simulink model "Lab1_3rev2022A"  (R2022a)
settings: Solver=ode23tb  StartTime=0.0  StopTime=3  RelTol=1e-3
values from neighbouring files (symbols this model uses):
  ki = 700    [script1_3 (1).m]    (also in script1_3.m)
  kii = 600    [script1_3 (1).m]    (also in script1_3.m)
  kiv = 0.077471    [script1_3 (1).m]    (also in script1_3.m)
  kp = 2.93    [script1_3 (1).m]    (also in script1_3.m)
  kpi = 4    [script1_3 (1).m]    (also in script1_3.m)
  kpv = 0.0011508    [script1_3 (1).m]    (also in script1_3.m)
  L = 2e-3    (= 0.002)    [script1_3 (1).m]    (also in script1_3.m)
  w_ref = 2*pi*60    (= 376.991118431)    [script1_3 (1).m]    (also in script1_3.m)
libraries: spsIGBTDiodeLib x6, spsSeriesRLCBranchLib x4, simulink x3, spsPWMGenerator2LevelLib x3, spsdq0toabcLib x3, spsabctodq0Lib x2, spsPVArrayLib x1, spsPower3phInstantaneousLib x1, spsThreePhaseVIMeasurementLib x1, spsThreePhaseSourceLib x1, spsVoltageMeasurementLib x1, spspowerguiLib x1
settings Model: Creator=Daniel  LastModifiedBy=Daniel

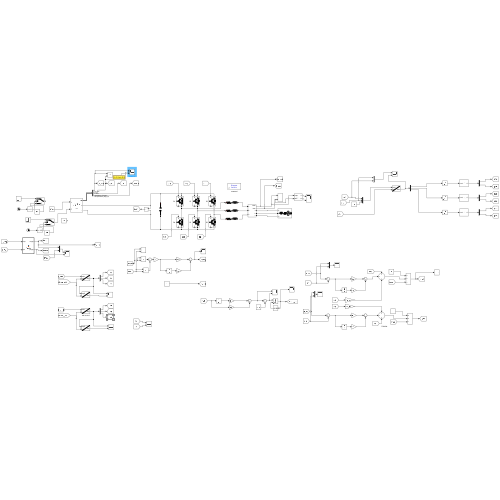
[thumbnail: Simulink's stored preview of the top-level diagram]
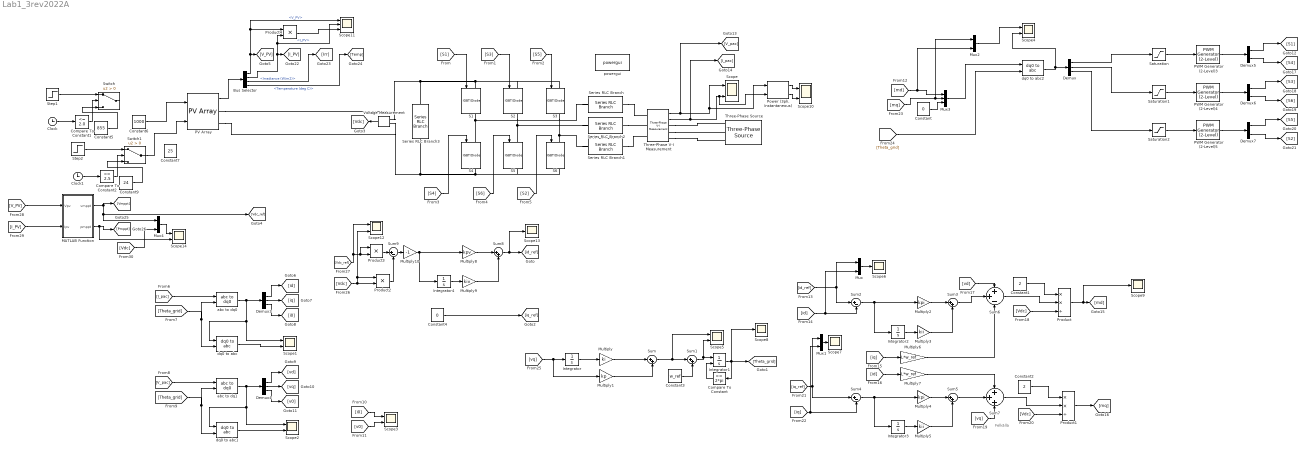
== system Lab1_3rev2022A ==
  note: Felkälla
  Bus Selector : BusSelector  OutputSignals=V_PV,I_PV,Irradiance (W/m2),Temperature (deg C)
  Clock : Clock
  Clock1 : Clock
  Compare To Constant : simulink/Logic and Bit Operations/Compare To Constant  relop=>=  const=2*pi  OutDataTypeStr=boolean
  Compare To Constant1 : simulink/Logic and Bit Operations/Compare To Constant  relop=<=  const=2.0  OutDataTypeStr=boolean
  Compare To Constant2 : simulink/Logic and Bit Operations/Compare To Constant  relop=<=  const=2.5  OutDataTypeStr=boolean
  Constant : Constant  Value=0
  Constant1 : Constant  Value=2
  Constant2 : Constant  Value=2
  Constant3 : Constant  Value=w_ref
  Constant4 : Constant  Value=0
  Constant5 : Constant  Value=855
  Constant6 : Constant  Value=1000
  Constant7 : Constant  Value=25
  Constant9 : Constant  Value=24
  Demux : Demux  Outputs=3
  Demux3 : Demux  Outputs=3
  Demux4 : Demux  Outputs=3
  Demux5 : Demux  Outputs=2
  Demux6 : Demux  Outputs=2
  Demux7 : Demux  Outputs=2
  Integrator{,2..4} (4 alike) : Integrator
  Integrator1 : Integrator  ExternalReset=rising
  MATLAB Function : MATLAB Function  TreatAsAtomicUnit=on
  Multiply : Gain  Gain=ki
  Multiply1 : Gain  Gain=kp
  Multiply10 : Gain  Gain=-1
  Multiply2 : Gain  Gain=kpi
  Multiply3 : Gain  Gain=kii
  Multiply4 : Gain  Gain=kpi
  Multiply5 : Gain  Gain=kii
  Multiply6 : Gain  Gain=L*w_ref
  Multiply7 : Gain  Gain=L*w_ref
  Multiply8 : Gain  Gain=kpv
  Multiply9 : Gain  Gain=kiv
  Mux{,1..2,4} (4 alike) : Mux  Inputs=2
  Mux3 : Mux  Inputs=3
  PV Array : spsPVArrayLib/PV Array  Npar=1  Nser=14  PlotType=array @ 1000 W/m2 & specified temperatures  S_vec="[ 1000  500  100 ]"  Temp_C_vec="[ 45 25  ]"  ModuleName=Trina Solar TSM-250PA05.08  PlotWhenSelected=off  Pm=249.86  Ncell=60  Voc=37.6  Isc=8.55  Vm=31  Im=8.06  beta_Voc_pc=-0.35  alpha_Isc_pc=0.06  beta_Voc=-0.1316  alpha_Isc=0.00513  IL=8.5795  I0=2.0381e-10  nI=0.99766  Rsh=301.8149  Rs=0.247  RobustModel=off  RobustCellTemperature=313.3991  BAL=on  Tc=1e-6  Tfilter=5e-5
  PWM Generator (2-Level)3 : spsPWMGenerator2LevelLib/PWM Generator (2-Level)  ModulatorType=Single-phase half-bridge (2 pulses)  ModulatorMode=Unsynchronized  Fc=20e3  Pc=90  nF=27  MinMax="[ -1  1 ]"  SamplingTechnique=Natural  ModulatingSignals=off  m=0.8  Freq=60  Phase=0  Ts=0  ShowCarrierOutport=off
  PWM Generator (2-Level)4 : spsPWMGenerator2LevelLib/PWM Generator (2-Level)  ModulatorType=Single-phase half-bridge (2 pulses)  ModulatorMode=Unsynchronized  Fc=20e3  Pc=90  nF=27  MinMax="[ -1  1 ]"  SamplingTechnique=Natural  ModulatingSignals=off  m=0.8  Freq=60  Phase=0  Ts=0  ShowCarrierOutport=off
  PWM Generator (2-Level)5 : spsPWMGenerator2LevelLib/PWM Generator (2-Level)  ModulatorType=Single-phase half-bridge (2 pulses)  ModulatorMode=Unsynchronized  Fc=20e3  Pc=90  nF=27  MinMax="[ -1  1 ]"  SamplingTechnique=Natural  ModulatingSignals=off  m=0.8  Freq=60  Phase=0  Ts=0  ShowCarrierOutport=off
  "Power (3ph, Instantaneous)" : spsPower3phInstantaneousLib/Power (3ph, Instantaneous)
  Product : Product  Inputs=**/
  Product1 : Product  Inputs=**/
  Product2 : Product
  Product3 : Product
  Product4 : Product
  S{1..6} (6 alike) : spsIGBTDiodeLib/IGBT//Diode  Ron=1e-3  Rs=1e5  Cs=inf  Measurements=on
  Saturation : Saturate  UpperLimit=1  LowerLimit=-1
  Saturation1 : Saturate  UpperLimit=1  LowerLimit=-1
  Saturation2 : Saturate  UpperLimit=1  LowerLimit=-1
  Scope{,1..5,10,12,14} (9 alike) : Scope  NumInputPorts=2
  Scope11 : Scope  NumInputPorts=3
  Scope{6..9,13} (5 alike) : Scope
  Series RLC Branch : spsSeriesRLCBranchLib/Series RLC Branch  LConnTagsString=__new0  RConnTagsString=__new0  BranchType=RL  Resistance=0.3  Inductance=2e-3  SetiL0=off  InitialCurrent=0  Capacitance=1e-6  Setx0=off  InitialVoltage=0  Measurements=None
  Series RLC Branch1 : spsSeriesRLCBranchLib/Series RLC Branch  LConnTagsString=__new0  RConnTagsString=__new0  BranchType=RL  Resistance=0.3  Inductance=2e-3  SetiL0=off  InitialCurrent=0  Capacitance=1e-6  Setx0=off  InitialVoltage=0  Measurements=None
  Series RLC Branch2 : spsSeriesRLCBranchLib/Series RLC Branch  LConnTagsString=__new0  RConnTagsString=__new0  BranchType=RL  Resistance=0.3  Inductance=2e-3  SetiL0=off  InitialCurrent=0  Capacitance=1e-6  Setx0=off  InitialVoltage=0  Measurements=None
  Series RLC Branch3 : spsSeriesRLCBranchLib/Series RLC Branch  LConnTagsString=__new0  RConnTagsString=__new0  BranchType=C  Resistance=1  Inductance=1e-3  SetiL0=off  InitialCurrent=0  Capacitance=4700e-6  Setx0=on  InitialVoltage=400  Measurements=None
  Step1 : Step  Before=1000  After=1200  SampleTime=0
  Step2 : Step  Time=1.5  Before=25  After=26.5  SampleTime=0
  Sum{,1,3,5,8} (5 alike) : Sum  Inputs=|++
  Sum2 : Sum  Inputs=|+-
  Sum4 : Sum  Inputs=|+-
  Sum6 : Sum  Inputs=++-
  Sum7 : Sum  Inputs=+++
  Sum9 : Sum  Inputs=|+-
  Switch : Switch  Criteria=u2 > Threshold  SaturateOnIntegerOverflow=off  InputSameDT=off
  Switch1 : Switch  Criteria=u2 > Threshold  SaturateOnIntegerOverflow=off  InputSameDT=off
  Three-Phase V-I Measurement : spsThreePhaseVIMeasurementLib/Three-Phase V-I Measurement  VoltageMeasurement=phase-to-ground  SetLabelV=off  LabelV=Vabc  Vpu=off  VpuLL=off  CurrentMeasurement=yes  SetLabelI=off  LabelI=Iabc  Ipu=off  Pbase=100e6  Vbase=500e3  OutputType=Complex  PhasorSimulation=off  PSBequivalent=0
  Three-Phase Source : spsThreePhaseSourceLib/Three-Phase Source  InternalConnection=Yg  VoltagePhases=off  Voltage=220  PhaseAngle=0  Voltage_phases=[25e3 25e3 25e3]/sqrt(3)  PhaseAngles_phases=[0 -120 +120]  Frequency=60  NonIdealSource=on  SpecifyImpedance=off  Resistance=0.3e-3  Inductance=1e-6  ShortCircuitLevel=100e6  BaseVoltage=220  XRratio=7  BusType=swing  Pref=10e3  Qref=0  Prefabc=[10e3, 10e3, 10e3]  Qrefabc=[0, 0, 0]  Qmin=-inf  Qmax=inf
  Voltage Measurement : spsVoltageMeasurementLib/Voltage Measurement  PhasorSimulation=off  OutputType=Complex  PSBequivalent=0
  abc to dq0 : spsabctodq0Lib/abc to dq0  Alignment=90 degrees behind phase A axis
  abc to dq1 : spsabctodq0Lib/abc to dq0  Alignment=90 degrees behind phase A axis
  dq0 to abc : spsdq0toabcLib/dq0 to abc  Alignment=90 degrees behind phase A axis
  dq0 to abc1 : spsdq0toabcLib/dq0 to abc  Alignment=90 degrees behind phase A axis
  dq0 to abc2 : spsdq0toabcLib/dq0 to abc  Alignment=90 degrees behind phase A axis
  powergui : spspowerguiLib/powergui  Priority=1  SimulationMode=Discrete  SampleTime=2e-6  frequency=60  Iterations=50  frequencyindice=0  Pbase=100e6  ErrMax=1e-4  UnitsV=kV  UnitsW=MW  buscounter=0  FunctionMessages=off  echomessages=off  EnableUseOfTLC=off  CurrentSourceSwitches=off  DisableSnubberDevices=off  DisableRonSwitches=off  DisableVfSwitches=off  DisplayEquations=off  AutomaticDiscreteSolvers=off  SolverType=Tustin/Backward Euler (TBE)  Interpol=off  ExternalGateDelay=off  methode=off  Ts=100  x0status=blocks  SPID=on  SwTol=0  HookPort=off  NonlinearTolerance=1e-4  nMaxIteration=100  ContinueOnMaxIteration=off  RestoreLinks=warning  ResistiveCurrentMeasurement=off  Frange=[0:2:500]  Ylog=off  Xlog=on  ShowGrid=off  save=off  variable=ZData  structure=0  ZoomFFT=off  StartTime=0.0  cycles=1  DisplayStyle=1  fundamental=60  FreqAxis=off  MaxFrequency=1000  frequencyindicesteady=1  RmsSteady=1  display=off
  wires:
  [S1] -> S1/1
  [S3] -> S2/1
  Three-Phase V-I Measurement/1 -> [V_pac], "Power (3ph, Instantaneous)"/1, Scope/1
  Three-Phase V-I Measurement/2 -> [I_pac], "Power (3ph, Instantaneous)"/2, Scope/2
  [S5] -> S3/1
  [S4] -> S4/1
  [S6] -> S5/1
  [S2] -> S6/1
  [I_pac] -> abc to dq0/1
  [Theta_grid] -> dq0 to abc/2, abc to dq0/2
  abc to dq0/1 -> Scope1/1, dq0 to abc/1, Demux3/1
  Demux3/1 -> [id]
  Demux3/2 -> [iq]
  Demux3/3 -> [i0]
  dq0 to abc/1 -> Scope1/2
  Demux4/3 -> [v0]
  Demux4/2 -> [vq]
  Demux4/1 -> [vd]
  [Theta_grid] -> dq0 to abc1/2, abc to dq1/2
  dq0 to abc1/1 -> Scope2/2
  [V_pac] -> abc to dq1/1
  abc to dq1/1 -> Scope2/1, dq0 to abc1/1, Demux4/1
  [i0] -> Scope3/1
  [v0] -> Scope3/2
  Mux/1 -> Scope6/1
  Integrator2/1 -> Multiply3/1
  Sum2/1 -> Integrator2/1, Multiply2/1
  Multiply2/1 -> Sum3/1
  Multiply3/1 -> Sum3/2
  Multiply5/1 -> Sum5/2
  Integrator3/1 -> Multiply5/1
  Sum4/1 -> Integrator3/1, Multiply4/1
  Multiply4/1 -> Sum5/1
  [id_ref] -> Sum2/1, Mux/1
  [id] -> Sum2/2, Mux/2
  [iq] -> Multiply6/1
  [id] -> Multiply7/1
  Sum3/1 -> Sum6/2
  Multiply6/1 -> Sum6/3
  [vd] -> Sum6/1
  Constant1/1 -> Product/1
  Sum6/1 -> Product/2
  [Vdc] -> Product/3
  Product/1 -> Scope9/1, [md]
  Multiply7/1 -> Sum7/1
  Sum5/1 -> Sum7/2
  [vq] -> Sum7/3
  Product1/1 -> [mq]
  Constant2/1 -> Product1/1
  Sum7/1 -> Product1/2
  [Vdc] -> Product1/3
  Mux1/1 -> Scope7/1
  [iq_ref] -> Sum4/1, Mux1/1
  [iq] -> Sum4/2, Mux1/2
  Demux5/2 -> [S4]
  Saturation/1 -> PWM Generator (2-Level)3/1
  PWM Generator (2-Level)3/1 -> Demux5/1
  Demux7/2 -> [S2]
  Saturation2/1 -> PWM Generator (2-Level)5/1
  PWM Generator (2-Level)4/1 -> Demux6/1
  Demux7/1 -> [S5]
  Demux5/1 -> [S1]
  Demux6/2 -> [S6]
  PWM Generator (2-Level)5/1 -> Demux7/1
  Saturation1/1 -> PWM Generator (2-Level)4/1
  Demux6/1 -> [S3]
  Demux/1 -> Saturation/1
  Demux/2 -> Saturation1/1
  Demux/3 -> Saturation2/1
  dq0 to abc2/1 -> Scope4/2, Demux/1
  Mux2/1 -> Scope4/1
  Constant/1 -> Mux3/3
  [md] -> Mux2/2, Mux3/1
  [mq] -> Mux2/1, Mux3/2
  Compare To Constant/1 -> Integrator1/2
  Integrator1/1 -> Compare To Constant/1, [Theta_grid], Scope8/1
  Constant3/1 -> Sum1/2
  Sum1/1 -> Integrator1/1, Scope5/2
  Multiply/1 -> Sum/1
  Sum/1 -> Scope5/1, Sum1/1
  Multiply1/1 -> Sum/2
  Integrator/1 -> Multiply/1
  [vq] -> Multiply1/1, Integrator/1
  [Theta_grid] -> dq0 to abc2/2
  Mux3/1 -> dq0 to abc2/1
  Voltage Measurement/1 -> [Vdc]
  "Power (3ph, Instantaneous)"/2 -> Scope10/2
  "Power (3ph, Instantaneous)"/1 -> Scope10/1
  Constant4/1 -> [iq_ref]
  Integrator4/1 -> Multiply9/1
  Multiply9/1 -> Sum8/2
  Multiply10/1 -> Integrator4/1, Multiply8/1
  Multiply8/1 -> Sum8/1
  Sum8/1 -> Scope13/1, [id_ref]
  Sum9/1 -> Multiply10/1
  Product2/1 -> Sum9/2
  Product3/1 -> Sum9/1
  [Vdc_ref] -> Scope12/1, Product3/1, Product3/2
  [Vdc] -> Product2/2, Product2/1, Scope12/2
  MATLAB Function/1(vmppt) -> [Vmppt], [Vdc_ref], Mux4/1
  PV Array/1 -> Bus Selector/1
  Bus Selector/1 -> Scope11/1, Product4/1, [V_PV]  "<V_PV>"
  Bus Selector/2 -> Scope11/2, Product4/2, [I_PV]  "<I_PV>"
  Bus Selector/3 -> [Irr]  "<Irradiance (W/m2)>"
  Bus Selector/4 -> [Temp]  "<Temperature (deg C)>"
  Product4/1 -> Scope11/3
  Step1/1 -> Switch/1
  Clock/1 -> Compare To Constant1/1
  Compare To Constant1/1 -> Switch/2
  Constant5/1 -> Switch/3
  Compare To Constant2/1 -> Switch1/2
  Constant9/1 -> Switch1/3
  Clock1/1 -> Compare To Constant2/1
  Step2/1 -> Switch1/1
  [V_PV] -> MATLAB Function/1(Vpv)
  [I_PV] -> MATLAB Function/2(Ipv)
  MATLAB Function/2(pmppt) -> Scope14/2, [Pmppt]
  [Vdc] -> Mux4/2
  Mux4/1 -> Scope14/1
  Constant6/1 -> PV Array/1
  Switch1/1 -> PV Array/2
  connections:
  PV Array/RConn1 -- Voltage Measurement/LConn1 -- Series RLC Branch3/LConn1 -- S3/LConn1 -- S2/LConn1 -- S1/LConn1
  PV Array/RConn2 -- Voltage Measurement/LConn2 -- Series RLC Branch3/RConn1 -- S6/RConn1 -- S5/RConn1 -- S4/RConn1
  S1/RConn1 -- Series RLC Branch/LConn1 -- S4/LConn1
  S2/RConn1 -- S5/LConn1 -- Series RLC Branch2/LConn1
  S3/RConn1 -- Series RLC Branch1/LConn1 -- S6/LConn1
  Series RLC Branch/RConn1 -- Three-Phase V-I Measurement/LConn1
  Series RLC Branch1/RConn1 -- Three-Phase V-I Measurement/LConn3
  Series RLC Branch2/RConn1 -- Three-Phase V-I Measurement/LConn2
  Three-Phase V-I Measurement/RConn1 -- Three-Phase Source/RConn1
  Three-Phase V-I Measurement/RConn2 -- Three-Phase Source/RConn2
  Three-Phase V-I Measurement/RConn3 -- Three-Phase Source/RConn3

== matlab function Lab1_3rev2022A/MATLAB Function ==
  data: Vpv input; vmppt output; Ipv input; pmppt output
function [ vmppt , pmppt ] = PandO ( Vpv , Ipv )
persistent Pold Vold vref
if isempty ( Vold )
    Vold = 0;
end
if isempty ( Pold )
    Pold = 0;
end
if isempty ( vref )
    vref = 434;
end
dV = 0.001;
P = Vpv * Ipv ;
if ( P ~= Pold )
    if (P > Pold )
        if ( Vpv > Vold )
            vref = vref + dV ;
        else
            vref = vref - dV ;
        end
        if (P < Pold )
            if ( Vpv > Vold )
                vref = vref - dV ;
            else
                vref = vref + dV ;
            end
        end
    end
end
Vold = Vpv ;
Pold = P ;
vmppt = vref ;
pmppt = P ;
